simulink library "Chassis_Axle3"  (R2025b)
settings: Solver=VariableStepAuto  StartTime=0.0  StopTime=10.0  RelTol=1e-3
undefined symbols (not defined in the file): Init, Vehicle
libraries: Tire_1x2x x6, Suspension x3, Aero_Coefficients x1, Body_Axle3 x1, Dampers_Axle3 x1, Springs_Axle3 x1
Description:
  | Copyright 2021-2025 The MathWorks, Inc.
settings Model: Creator=smiller  LastModifiedBy=smiller
settings SolverCC: AlgebraicLoopSolver=TrustRegion
settings DataIOCC: ReturnWorkspaceOutputs=off
settings DebuggingCC: UnconnectedInputMsg=warning  UnconnectedOutputMsg=warning  UnconnectedLineMsg=warning  ArithmeticOperatorsInVariantConditions=warning
settings ModelReferenceCC: EnableRefExpFcnMdlSchedulingChecks=on
settings SFSimCC: CustomCodeUndefinedFunction=UseInterfaceOnly
settings RTWCC: GPUComputeCapability=3.5  DLArmComputeVersion=19.05

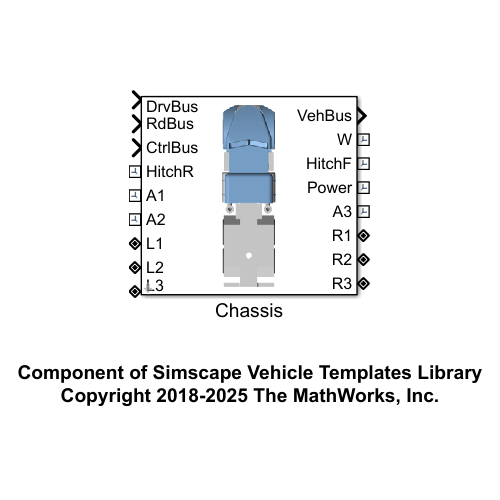
[thumbnail: Simulink's stored preview of the top-level diagram]
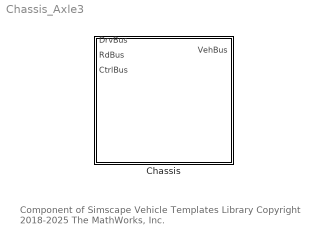
== system Chassis_Axle3 ==
  note: Component of Simscape Vehicle Templates Library
      | Copyright 2018-2025 The MathWorks, Inc.
  Chassis : Subsystem  Tag=PublishSubsystem  VariantControl=Chassis  mask(Chassis){Chassis=Vehicle.Chassis, Init=Init, mask_image_name=sm_car_vehicle_chassis_custom_IMAGE.png, veh_index=1}
      mask prompts: Chassis "Vehicle Parameters"; Init "Initial Values"; mask_image_name "Mask Image (string)"; veh_index "Vehicle Index (for tires)"
      mask help: Models vehicle chassis, with suspension, body, tires, springs, and dampers.
      mask Help: web('sm_car_doc_chassis.html')
      mask Display:
      | % Get image from BodyGeometry.class
      | % (active choice for Body Geometry subsystem)
      | temp_veh_bg_class = lower(get_param([gcb '/Body/Body Geometry'],'LabelModeActiveChoice'));
      | 
      | imagestr = (['sm_car_chassis_' temp_veh_bg_class '.png']);
      | if(~exist(imagestr))
      |     imagestr = ['sm_car_chassis_default.png'];
      | end
      | 
      | image(imagestr);

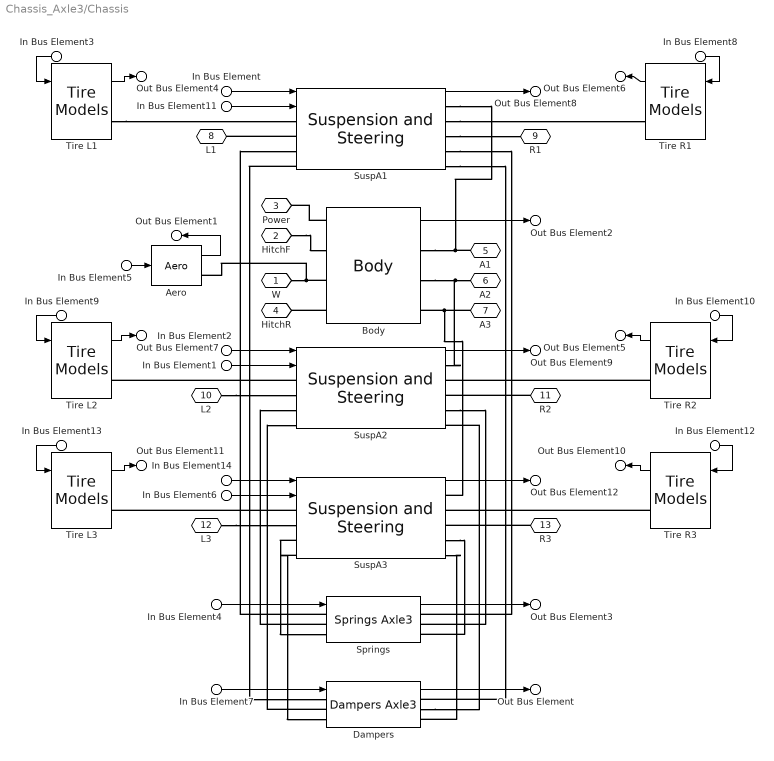
== system Chassis_Axle3/Chassis ==
  In Bus Element11 : Inport  PortName=DrvBus
  In Bus Element1 : Inport  PortName=DrvBus
  In Bus Element6 : Inport  PortName=DrvBus
  In Bus Element3 : Inport  Port=2  PortName=RdBus  Element=L1
  In Bus Element8 : Inport  Port=2  PortName=RdBus  Element=R1
  In Bus Element10 : Inport  Port=2  PortName=RdBus  Element=R2
  In Bus Element9 : Inport  Port=2  PortName=RdBus  Element=L2
  In Bus Element5 : Inport  Port=2  PortName=RdBus  Element=fWindCar
  In Bus Element12 : Inport  Port=2  PortName=RdBus  Element=R3
  In Bus Element13 : Inport  Port=2  PortName=RdBus  Element=L3
  In Bus Element7 : Inport  Port=3  PortName=CtrlBus  Element=Damper
  In Bus Element : Inport  Port=3  PortName=CtrlBus  Element=SuspA1
  In Bus Element4 : Inport  Port=3  PortName=CtrlBus  Element=Spring
  In Bus Element2 : Inport  Port=3  PortName=CtrlBus  Element=SuspA2
  In Bus Element14 : Inport  Port=3  PortName=CtrlBus  Element=SuspA3
  Aero : Aero_Coefficients/Aero  CL=Chassis.Aero.CL.Value  CD=Chassis.Aero.CD.Value  rho=Chassis.Aero.rho_air.Value  A=Chassis.Aero.ARef.Value  sCentreOfPressure=Chassis.Aero.sPressureCentre.Value  clr_hp=Visual.hp.clr  opc_hp=Visual.hp.opc  rad_hp=Visual.hp.rad
  Body : Body_Axle3/Body  hp_mount_a1=Chassis.Body.sAxle1.Value  hp_mount_a2=Chassis.Body.sAxle2.Value  hp_mount_a3=Chassis.Body.sAxle3.Value  hp_mount_power=Chassis.Body.sPower.Value  hp_chassis_cg=Chassis.Body.sCG.Value  hp_mount_hitchf=Chassis.Body.sHitchF.Value  hp_mount_hitchr=Chassis.Body.sHitchR.Value  chassis_mass=Chassis.Body.m.Value  chassis_inertia=Chassis.Body.J.Value  clr_chassis_hp_cg=Visual.hp.clr  opc_chassis_hp_cg=Visual.hp.opc  size_chassis_hp_cg=Visual.hp.rad  BodyGeometry=Chassis.Body.BodyGeometry  Passenger=Chassis.Body.Passenger
  Dampers : Dampers_Axle3/Dampers Axle3  VariantControl=Variant1  LabelModeActiveChoice=Independent  Damper=Vehicle.Chassis.Damper  VariantLabel=Vehicle.Chassis.Damper.class.Value
      settings: AttributesFormatString=%<ActiveVariant>
  Springs : Springs_Axle3/Springs Axle3  VariantControl=Variant1  LabelModeActiveChoice=Independent  Spring=Vehicle.Chassis.Spring  VariantLabel=Vehicle.Chassis.Spring.class.Value
      settings: AttributesFormatString=%<ActiveVariant>
  SuspA1 : Suspension/Suspension and Steering  VariantControl=Variant1  LabelModeActiveChoice=Linkage  Susp=Chassis.SuspA1  Init=Init.Axle1  VariantLabel=Chassis.SuspA1.class.Value
      settings: AttributesFormatString=%<LabelModeActiveChoice>
  SuspA2 : Suspension/Suspension and Steering  VariantControl=Variant1  LabelModeActiveChoice=Linkage  Susp=Chassis.SuspA2  Init=Init.Axle2  VariantLabel=Chassis.SuspA2.class.Value
      settings: AttributesFormatString=%<LabelModeActiveChoice>
  SuspA3 : Suspension/Suspension and Steering  VariantControl=Variant1  LabelModeActiveChoice=Simple  Susp=Chassis.SuspA3  Init=Init.Axle3  VariantLabel=Chassis.SuspA3.class.Value
      settings: AttributesFormatString=%<LabelModeActiveChoice>
  Tire L1 : Tire_1x2x/Tire Models  Tag=PublishSubsystem  VariantControl=Variant1  LabelModeActiveChoice=MFMbody  popup_leftRight=Left  tir_index=veh_index  Tire=Chassis.TireA1  VariantLabel=Chassis.TireA1.class.Value
      settings: AttributesFormatString=%<ActiveVariant>
  Tire L2 : Tire_1x2x/Tire Models  Tag=PublishSubsystem  VariantControl=Variant1  LabelModeActiveChoice=MFMbody  popup_leftRight=Left  tir_index=veh_index+10  Tire=Chassis.TireA2  VariantLabel=Chassis.TireA2.class.Value
      settings: AttributesFormatString=%<ActiveVariant>
  Tire L3 : Tire_1x2x/Tire Models  Tag=PublishSubsystem  VariantControl=Variant1  LabelModeActiveChoice=Tire2x  popup_leftRight=Left  tir_index=veh_index+20  Tire=Chassis.TireA3  VariantLabel=Chassis.TireA3.class.Value
      settings: AttributesFormatString=%<ActiveVariant>
  Tire R1 : Tire_1x2x/Tire Models  Tag=PublishSubsystem  VariantControl=Variant1  LabelModeActiveChoice=MFMbody  popup_leftRight=Right  tir_index=veh_index+4  Tire=Chassis.TireA1  VariantLabel=Chassis.TireA1.class.Value
      settings: AttributesFormatString=%<ActiveVariant>
  Tire R2 : Tire_1x2x/Tire Models  Tag=PublishSubsystem  VariantControl=Variant1  LabelModeActiveChoice=MFMbody  popup_leftRight=Right  tir_index=veh_index+14  Tire=Chassis.TireA2  VariantLabel=Chassis.TireA2.class.Value
      settings: AttributesFormatString=%<ActiveVariant>
  Tire R3 : Tire_1x2x/Tire Models  Tag=PublishSubsystem  VariantControl=Variant1  LabelModeActiveChoice=Tire2x  popup_leftRight=Right  tir_index=veh_index+24  Tire=Chassis.TireA3  VariantLabel=Chassis.TireA3.class.Value
      settings: AttributesFormatString=%<ActiveVariant>
  W : PMIOPort  Side=Right
  HitchF : PMIOPort  Port=2  Side=Right
  Power : PMIOPort  Port=3  Side=Right
  HitchR : PMIOPort  Port=4  Side=Left
  A1 : PMIOPort  Port=5  Side=Left
  A2 : PMIOPort  Port=6  Side=Left
  A3 : PMIOPort  Port=7  Side=Right
  L1 : PMIOPort  Port=8  Side=Left
  R1 : PMIOPort  Port=9  Side=Right
  L2 : PMIOPort  Port=10  Side=Left
  R2 : PMIOPort  Port=11  Side=Right
  L3 : PMIOPort  Port=12  Side=Left
  R3 : PMIOPort  Port=13  Side=Right
  Out Bus Element4 : Outport  VectorParamsAs1DForOutWhenUnconnected=off  PortName=VehBus  Element=WhlL1
  Out Bus Element6 : Outport  VectorParamsAs1DForOutWhenUnconnected=off  PortName=VehBus  Element=WhlR1
  Out Bus Element5 : Outport  VectorParamsAs1DForOutWhenUnconnected=off  PortName=VehBus  Element=WhlR2
  Out Bus Element7 : Outport  VectorParamsAs1DForOutWhenUnconnected=off  PortName=VehBus  Element=WhlL2
  Out Bus Element1 : Outport  VectorParamsAs1DForOutWhenUnconnected=off  PortName=VehBus  Element=Aero
  Out Bus Element : Outport  VectorParamsAs1DForOutWhenUnconnected=off  PortName=VehBus  Element=Damper
  Out Bus Element3 : Outport  VectorParamsAs1DForOutWhenUnconnected=off  PortName=VehBus  Element=Spring
  Out Bus Element8 : Outport  VectorParamsAs1DForOutWhenUnconnected=off  PortName=VehBus  Element=SuspA1
  Out Bus Element9 : Outport  VectorParamsAs1DForOutWhenUnconnected=off  PortName=VehBus  Element=SuspA2
  Out Bus Element2 : Outport  VectorParamsAs1DForOutWhenUnconnected=off  PortName=VehBus  Element=Body
  Out Bus Element10 : Outport  VectorParamsAs1DForOutWhenUnconnected=off  PortName=VehBus  Element=WhlR3
  Out Bus Element11 : Outport  VectorParamsAs1DForOutWhenUnconnected=off  PortName=VehBus  Element=WhlL3
  Out Bus Element12 : Outport  VectorParamsAs1DForOutWhenUnconnected=off  PortName=VehBus  Element=SuspA3
  wires:
  Body/1 -> Out Bus Element2/1
  In Bus Element5/1 -> Aero/1
  Aero/1 -> Out Bus Element1/1
  In Bus Element4/1 -> Springs/1
  In Bus Element7/1 -> Dampers/1
  In Bus Element2/1 -> SuspA2/1
  SuspA2/1 -> Out Bus Element9/1
  In Bus Element1/1 -> SuspA2/2
  In Bus Element/1 -> SuspA1/1
  SuspA1/1 -> Out Bus Element8/1
  In Bus Element11/1 -> SuspA1/2
  Tire R2/1 -> Out Bus Element5/1
  In Bus Element9/1 -> Tire L2/1
  Tire L1/1 -> Out Bus Element4/1
  In Bus Element8/1 -> Tire R1/1
  Tire L2/1 -> Out Bus Element7/1
  In Bus Element10/1 -> Tire R2/1
  Tire R1/1 -> Out Bus Element6/1
  In Bus Element3/1 -> Tire L1/1
  Dampers/1 -> Out Bus Element/1
  Springs/1 -> Out Bus Element3/1
  In Bus Element12/1 -> Tire R3/1
  Tire L3/1 -> Out Bus Element11/1
  In Bus Element13/1 -> Tire L3/1
  Tire R3/1 -> Out Bus Element10/1
  In Bus Element6/1 -> SuspA3/2
  SuspA3/1 -> Out Bus Element12/1
  In Bus Element14/1 -> SuspA3/1
  connections:
  Body/LConn4 -- HitchR/RConn1
  Body/LConn1 -- Power/RConn1
  Dampers/RConn2 -- SuspA2/RConn5
  Dampers/LConn2 -- SuspA2/LConn4
  SuspA2/RConn4 -- Springs/RConn2
  Springs/LConn2 -- SuspA2/LConn3
  R2/RConn1 -- SuspA2/RConn3
  L2/RConn1 -- SuspA2/LConn2
  Tire R2/RConn1 -- SuspA2/RConn2
  SuspA2/LConn1 -- Tire L2/RConn1
  SuspA1/RConn5 -- Dampers/RConn1
  SuspA1/LConn4 -- Dampers/LConn1
  SuspA1/RConn4 -- Springs/RConn1
  Springs/LConn1 -- SuspA1/LConn3
  SuspA1/RConn1 -- Body/RConn1 -- A1/RConn1
  Tire L1/RConn1 -- SuspA1/LConn1
  SuspA1/RConn2 -- Tire R1/RConn1
  SuspA1/RConn3 -- R1/RConn1
  SuspA1/LConn2 -- L1/RConn1
  A2/RConn1 -- Body/RConn2 -- SuspA2/RConn1
  W/RConn1 -- Body/LConn3 -- Aero/RConn1
  SuspA3/LConn1 -- Tire L3/RConn1
  Tire R3/RConn1 -- SuspA3/RConn2
  L3/RConn1 -- SuspA3/LConn2
  R3/RConn1 -- SuspA3/RConn3
  A3/RConn1 -- Body/RConn3 -- SuspA3/RConn1
  SuspA3/LConn3 -- Springs/LConn3
  SuspA3/RConn4 -- Springs/RConn3
  SuspA3/RConn5 -- Dampers/RConn3
  SuspA3/LConn4 -- Dampers/LConn3
  HitchF/RConn1 -- Body/LConn2
